simulink model "receiver"  (R2013b)
settings: Solver=FixedStepDiscrete  SolverMode=SingleTasking  StartTime=0  StopTime=8000  RelTol=1e-3
model workspace (MAT data in the model file):
  logicAddr = 2
settings Model: Creator=qiji  LastModifiedBy=qiji
settings DataIOCC: SaveOutput=off  SaveTime=off
settings OptimizationCC: BlockReduction=off  ConditionallyExecuteInputs=off  InlineParams=on
settings DebuggingCC: UnderspecifiedInitializationDetection=Simplified  MultiTaskDSMMsg=warning  MultiTaskCondExecSysMsg=none  SingleTaskRateTransMsg=error  SFUnusedDataAndEventsDiag=none
settings RTWCC: IncludeERTFirstTime=on
settings GRTTargetCC: CodeReplacementLibrary=None  CPPClassGenCompliant=on
settings ConfigurationSet: Description=SimMechanics 2G

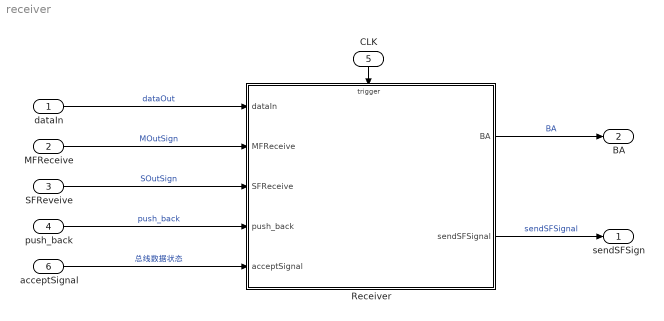
== system receiver ==
  dataIn : Inport  OutDataTypeStr=uint32  PortDimensions=1  SampleTime=[1,0]
  "MFReceive " : Inport  Port=2  OutDataTypeStr=boolean  PortDimensions=1  SampleTime=[1,0]
  SFReveive : Inport  Port=3  OutDataTypeStr=boolean  PortDimensions=1  SampleTime=[1,0]
  push_back : Inport  Port=4  OutDataTypeStr=boolean  PortDimensions=1  SampleTime=[1,0]
  CLK : Inport  Port=5  OutDataTypeStr=boolean  PortDimensions=1  SampleTime=[1,0]
  acceptSignal : Inport  Port=6  OutDataTypeStr=uint8  PortDimensions=1  SampleTime=[1,0]
  Receiver : Stateflow chart  TreatAsAtomicUnit=on
  sendSFSign : Outport  OutDataTypeStr=uint8  PortDimensions=1  SampleTime=[1,0]
  BA : Outport  Port=2  OutDataTypeStr=boolean  PortDimensions=1  SampleTime=[1,0]
  wires:
  Receiver/1(BA) -> BA/1  "BA"
  Receiver/2(sendSFSignal) -> sendSFSign/1  "sendSFSignal"
  acceptSignal/1 -> Receiver/5(acceptSignal)  "总线数据状态"
  push_back/1 -> Receiver/4(push_back)  "push_back"
  dataIn/1 -> Receiver/1(dataIn)  "dataOut"
  SFReveive/1 -> Receiver/3(SFReceive)  "SOutSign"
  "MFReceive "/1 -> Receiver/2(MFReceive)  "MOutSign"
  CLK/1 -> Receiver/Trigger

== stateflow chart receiver/Receiver ==
  settings: sampleTime=4.1666666667e-8  executeAtInitialization=1  initializeOutput=1
  state receiveMF [parallel]
    settings: executionOrder=1
    state wait
      en:
      [buffer, BufferIndex]= initBuffer();
    state wait4MFEnd
    state judgeAddr
    state MFReceive
    state MFcode0
    state MFcode8
    state MFcode15
    state MTrans
    note: 如果收到了f_code为15的主帧，则应该获得主权
    (default) -> receiveMF.wait
    judgeAddr -> receiveMF.wait [order 2]
    MTrans -> receiveMF.wait
    receiveMF.wait -> wait4MFEnd : [MFReceive==true]
    wait4MFEnd -> judgeAddr : [MFReceive == false]
        | {fcodeIn = uint8(getFCode(buffer));
        | addrIn = uint16(getAddr(buffer));
        | }
    judgeAddr -> MFReceive [order 1] : [addrIn == LogicAddr]
    MFReceive -> MFcode0 [order 2] : [fcodeIn == 0]
    MFReceive -> MFcode8 [order 3] : [fcodeIn == 8]
    MFReceive -> MFcode15 [order 1] : [fcodeIn == 15 ]
    MFcode0 -> MTrans : {sendSFSignal=1;}
    MFcode8 -> MTrans : {sendSFSignal=2;}
    MFcode15 -> MTrans : {sendSFSignal=3;
        | BAPrepare = true;}
  state receiveSF1 [parallel]
    settings: executionOrder=3
    note: acceptSF, acceptACT, acceptDomain在发送完主帧以后，根据主帧的类型进行相应的置位
        | 收到fcode为8的从帧之后，说明目标设备已经返回了OK，这时应该将BA置位
    state wait
      en:
      initBuffer();
      temp=0;
    state wait4SF
    state wait4ACT
    state wait4Domain
    state wait4SFEnd
    state test
    state STrans
    (default) -> receiveSF1.wait
    (junction 268) -> receiveSF1.wait : {
        | BufferIndex = 0;
        | }
    receiveSF1.wait -> (junction 268) [order 4] : [SFReceive == true]
        | {BA = getBA(BAPrepare)
        | BAPrepare = false;}
    receiveSF1.wait -> wait4SF [order 1] : [acceptSignal == 1]
        | {
        | temp=1;
        | }
    receiveSF1.wait -> wait4ACT [order 2] : [acceptSignal==2]
        | {
        | temp=2;
        | }
    receiveSF1.wait -> wait4Domain [order 3] : [acceptSignal==3]
        | {
        | temp=3;
        | }
    wait4SF -> wait4SFEnd : [SFReceive == true]
    wait4ACT -> wait4SFEnd : [SFReceive==true]
    wait4Domain -> wait4SFEnd : [SFReceive==true]
    test -> (junction 268) [order 2]
    STrans -> (junction 268) : [SFReceive == false]
        | {
        | BA = reset(temp);
        | }
    wait4SFEnd -> test : [SFReceive == false]
    test -> STrans [order 1] : [judge(temp, buffer)]
  state Buffer [parallel]
    settings: executionOrder=2
    state wait
    state push_back
      en:
      buffer[BufferIndex]=dataIn;
      BufferIndex = BufferIndex+1;
    (default) -> Buffer.wait : {
        | BufferIndex = uint8(0);
        | }
    Buffer.wait -> push_back : [push_back==1]
    push_back -> Buffer.wait
  data: tmp function_input uint8; r function_output boolean; prepare function_input boolean; r function_output boolean; tmp function_input uint8; data function_input uint16 size=16; r function_output boolean; temp local uint8; r function_output uint16 size=16; index function_output uint8; data function_input uint32; num function_input uint32; r function_output uint32; data function_input uint16 size=16; r function_output uint16; bit1 temporary uint16; bit2 temporary uint16; bit3 temporary uint16; bit0 temporary uint16; data function_input uint32; r function_output uint32; r function_output uint32; data function_input uint32; data function_input uint16 size=16; r function_output uint16; dataIn input uint32; MFReceive input boolean; SFReceive input boolean; fcodeIn local uint8; addrIn local uint16; BA output boolean; BufferIndex local uint8; buffer local uint16 size=16 =[0,0,0,0,0,0,0,0,0,0,0,0,0,0,0,0]; push_back input boolean; LogicAddr constant uint8 =2; sendSFSignal output uint8 =0; acceptSignal input uint8; BAPrepare local boolean
  events: CLK input RISING_EDGE_EVENT
  function r = reset(tmp):
    | function r = reset(tmp)
    | r = false;
    | if tmp==3
    |     r = true;
    | end;
  function r = getBA(prepare):
    | function r = getBA(prepare)
    | r = false;
    | if prepare == true
    |     r = true;
    | end;
  function r = judge(tmp, data):
    | function r = judge(tmp, data)
    | if tmp==1
    |     r = true;
    | elseif tmp==2 && bitget(data(2), 6)
    |     r = true;
    | elseif tmp==3 && bitget(data(2), 8)
    |     r = true;
    | else
    |     r = false;
    | end
  function [r, index] = initBuffer:
    | function [r, index] = initBuffer
    | r = [(uint16(0));(uint16(0));(uint16(0));(uint16(0));...
    |     (uint16(0));(uint16(0));(uint16(0));(uint16(0));...
    |     (uint16(0));(uint16(0));(uint16(0));(uint16(0));...
    |     (uint16(0));(uint16(0));(uint16(0));(uint16(0))];
    | index=uint8(0);
  function r = getbit(data, num):
    | function r = getbit(data, num)
    | r = bitget(uint32(data), num);
  function r = getFCode(data):
    | function r = getFCode(data)
    | bit0 = bitget(data(2), 9);
    | bit1 = bitget(data(2), 10);
    | bit2 = bitget(data(2), 11);
    | bit3 = bitget(data(2), 12);
    | r = bit0+bit1*2+bit2*4+bit3*8;
  function r = ManchesterEncoding(data):
    | function r = ManchesterEncoding(data)
    | r = data;
    | for i = 1:16
    |     x = bitget(data, i);
    |     if x == 0
    |         r = bitset(r, i*2-1, 1);
    |         r = bitset(r, i*2, 0);
    |     else
    |         r = bitset(r, i*2-1, 0);
    |         r = bitset(r, i*2, 1);
    |     end
    | end
  function r = ManchesterDecoding(data):
    | function r = ManchesterDecoding(data)
    | r = uint32(0);
    | for i = (1:2:32)
    |     x0 = bitget(data, i);
    |     x1 = bitget(data, i+1);
    |     if x0==0 && x1==1
    |         r = bitset(r, (i+1)/2, 1);
    |     else
    |         r = bitset(r, (i+1)/2, 0);
    |     end
    | end
  function r = getAddr(data):
    | function r = getAddr(data)
    | %取出buffer(2)后8位
    | high8 = bitshift(bitshift(uint16(data(2)), 8), -4);
    | % 取出buffer(3)前4位
    | low4 = bitshift(uint16(data(3)), -12);
    | r = high8 + low4;
